simulink model "StateSpace_Sim"  (R2018a)
settings: Solver=VariableStepAuto  StartTime=0.0  StopTime=10.0  RelTol=1e-3
values from neighbouring files (symbols this model uses):
  A = 1/JT*[ 0 0                          JT                    0 ... (first row only)    [InvPend_StateSpace.m]
  B = Kg*kt*etag*etam/Rm * B    [InvPend_StateSpace.m]
  C = zpk( z, p, k )    [InvPend_PID.m]    (also in InvPend_StateSpace.m = [ 1 0 0 0)
  K = 0.465    [InvPend_PID.m]    (also in InvPend_StateSpace.m = lqr( A, B, Q, R ))
  L = place( A', C', P )'    [InvPend_StateSpace.m]
  Nbar = rscale( sys_ss, K )    [InvPend_StateSpace.m]
libraries: dspsigattribs x1
settings Model: Creator=andrewchulock  LastModifiedBy=andrewchulock

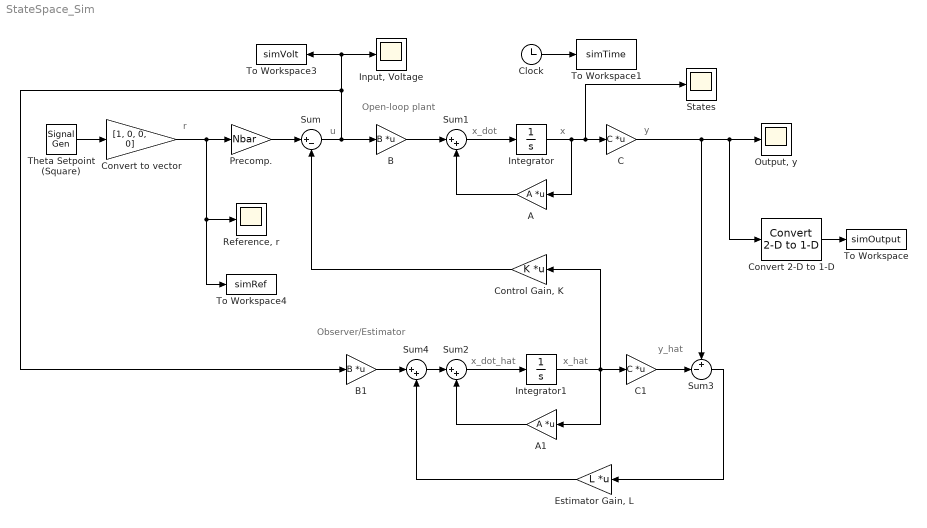
== system StateSpace_Sim ==
  note: Open-loop plant
  note: y
  note: x
  note: x_dot
  note: u
  note: r
  note: Observer/Estimator
  note: y_hat
  note: x_hat
  note: x_dot_hat
  A : Gain  Gain=A  Multiplication=Matrix(K*u)
  A1 : Gain  Gain=A  Multiplication=Matrix(K*u)
  B : Gain  Gain=B  Multiplication=Matrix(K*u)
  B1 : Gain  Gain=B  Multiplication=Matrix(K*u)
  C : Gain  Gain=C  Multiplication=Matrix(K*u)
  C1 : Gain  Gain=C  Multiplication=Matrix(K*u)
  Clock : Clock
  "Control Gain, K" : Gain  Gain=K  Multiplication=Matrix(K*u)
  Convert 2-D to 1-D : dspsigattribs/Convert 2-D to 1-D
      settings: SourceProductName=DSP System Toolbox  SourceProductBaseCode=DS
  Convert to vector : Gain  Gain=[1, 0, 0, 0]
  "Estimator Gain, L" : Gain  Gain=L  Multiplication=Matrix(K*u)
  "Input, Voltage" : Scope
  Integrator : Integrator
  Integrator1 : Integrator
  "Output, y" : Scope
  Precomp. : Gain  Gain=Nbar
  "Reference, r" : Scope
  States : Scope
  Sum : Sum  Inputs=|+-
  Sum1 : Sum  Inputs=|++
  Sum2 : Sum  Inputs=|++
  Sum3 : Sum  Inputs=+-|
  Sum4 : Sum  Inputs=|++
  Theta Setpoint (Square) : SignalGenerator  WaveForm=square  Amplitude=-0.35  Frequency=0.1
  To Workspace : ToWorkspace  VariableName=simOutput  SampleTime=-1
      settings: Save2DSignal=2-D array (concatenate along first dimension)
  To Workspace1 : ToWorkspace  VariableName=simTime  SampleTime=-1
      settings: Save2DSignal=2-D array (concatenate along first dimension)
  To Workspace3 : ToWorkspace  VariableName=simVolt  SampleTime=-1
      settings: Save2DSignal=2-D array (concatenate along first dimension)
  To Workspace4 : ToWorkspace  VariableName=simRef  SampleTime=-1
      settings: Save2DSignal=2-D array (concatenate along first dimension)
  wires:
  Convert to vector/1 -> Precomp./1, To Workspace4/1, "Reference, r"/1
  Precomp./1 -> Sum/1
  B/1 -> Sum1/1
  Sum1/1 -> Integrator/1
  Integrator/1 -> A/1, C/1, States/1
  A/1 -> Sum1/2
  C/1 -> Convert 2-D to 1-D/1, "Output, y"/1, Sum3/1
  "Control Gain, K"/1 -> Sum/2
  A1/1 -> Sum2/2
  Integrator1/1 -> "Control Gain, K"/1, A1/1, C1/1
  Sum/1 -> To Workspace3/1, "Input, Voltage"/1, B1/1, B/1
  Sum2/1 -> Integrator1/1
  C1/1 -> Sum3/2
  Sum4/1 -> Sum2/1
  B1/1 -> Sum4/1
  Sum3/1 -> "Estimator Gain, L"/1
  "Estimator Gain, L"/1 -> Sum4/2
  Clock/1 -> To Workspace1/1
  Convert 2-D to 1-D/1 -> To Workspace/1
  Theta Setpoint (Square)/1 -> Convert to vector/1
